simulink model "xpcFrameloop"  (Simulink 5.0)
settings: Solver=FixedStepDiscrete  StartTime=0.0  StopTime=10.0  RelTol=1e-3
libraries: dspsigattribs x2, xpclib x1, dspsrcs4 x1
settings Model: Creator=gweast  LastModifiedBy=gweast  ExtModeMexFile=ext_xpc  ExtModeArmWhenConnect=off  BooleanDataType=off  OptimizeBlockIOStorage=off  RTWSystemTargetFile=xpctarget.tlc  RTWTemplateMakefile=xpc_default_tmf  RTWOptions="-aEnforceIntegerDowncast=0 -aExtMode=1 -aFoldNonRolledExpr=0 -aForceParamTrailComments=0 -aGenerateComments=1 -aGenerateReport=0 -aIncDataTypeInIds=0 -aIncHierarchyInIds=0 -aInlineInvariantSignals=0 -aInlineParameters=0 -aInlinedPrmAccess=\"Literals\" -aLocalBlockOutputs=0 -aMaxRTWIdLen=31 -aPrefixModelToSubsysFcnNames=1 -aRL32IRQSourceModifier=\"Timer\" -aRL32LogBufSizeModifier=100000 -aRL32LogTETModifier=1 -aRL32ModeModifier=\"Real-Time\" -aRL32ObjectName=\"tg\" -aRTWVerbose=1 -aRollThreshold=5 -aShowEliminatedStatements=1 -axPCIOIRQSlot=-1 -axPCIRQSourceBoard=\"None/Other\" -axpcDblBuff=0 -axpcObjCom=0"

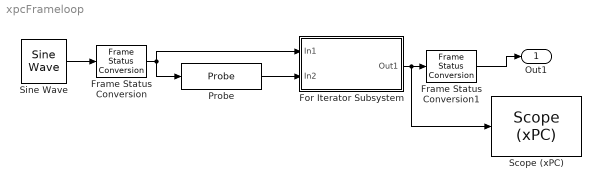
== system xpcFrameloop ==
  For Iterator Subsystem : Subsystem  TreatAsAtomicUnit=on
  Frame Status Conversion : dspsigattribs/Frame Status Conversion  growRefPort=off  outframe=Sample-based
  Frame Status Conversion1 : dspsigattribs/Frame Status Conversion  growRefPort=off  outframe=Frame-based
  Probe : Probe  ProbeSampleTime=off  ProbeComplexSignal=off
  "Scope (xPC) " : xpclib/Misc./Scope (xPC)   scopeno=1  scopetype=Target  viewmode=Graphical redraw  grid=on  ylimits=[0,0]  autostart=on  nosamples=100  noprepostsamples=0  interleave=1  triggermode=FreeRun  triggersignal=1  triggerlevel=0.0  triggerslope=either  triggerscope=1  triggersample=0
  Sine Wave : dspsrcs4/Sine Wave  Amplitude=1  Frequency=100  Phase=0  SampleMode=Discrete  OutComplex=Real  CompMethod=Trigonometric fcn  TableSize=Speed  SampleTime=1/1000  SamplesPerFrame=11  dataType=double  wordLen=16  udDataType=sfix(16)  fracBitsMode=Best precision  numFracBits=14  ResetState=Restart at time zero
  Out1 : Outport
  wires:
  Frame Status Conversion/1 -> For Iterator Subsystem/1(In1), Probe/1
  For Iterator Subsystem/1(Out1) -> Frame Status Conversion1/1, "Scope (xPC) "/1
  Frame Status Conversion1/1 -> Out1/1
  Probe/1 -> For Iterator Subsystem/2(In2)
  Sine Wave/1 -> Frame Status Conversion/1

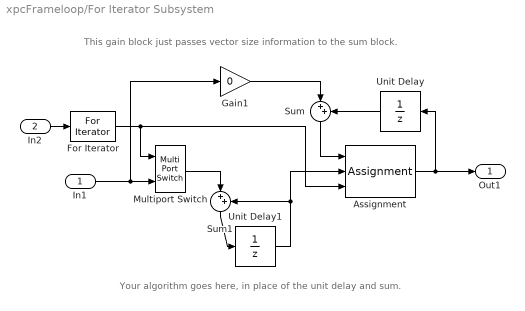
== system xpcFrameloop/For Iterator Subsystem ==
  note: Your algorithm goes here, in place of the
      | unit delay and sum.
  note: This gain block just passes vector
      | size information to the sum block.
  In1 : Inport
  In2 : Inport  Port=2
  Assignment : Assignment  ElementSrc=External
  For Iterator : ForIterator  IterationSource=external  NumIters=10
  Gain1 : Gain  Gain=0  SaturateOnIntegerOverflow=on
  Multiport Switch : MultiPortSwitch  Inputs=1  SaturateOnIntegerOverflow=on  InputSameDT=on
  Sum : Sum  Orientation=down  Inputs=|++  SaturateOnIntegerOverflow=on  InputSameDT=on
  Sum1 : Sum  Orientation=down  Inputs=|++  SaturateOnIntegerOverflow=on  InputSameDT=on
  Unit Delay : UnitDelay  Orientation=left  SampleTime=-1
  Unit Delay1 : UnitDelay  SampleTime=-1
  Out1 : Outport
  wires:
  For Iterator/1 -> Multiport Switch/1, Assignment/3
  In1/1 -> Multiport Switch/2, Gain1/1
  Assignment/1 -> Unit Delay/1, Out1/1
  Unit Delay1/1 -> Assignment/2, Sum1/2
  Unit Delay/1 -> Sum/2
  Sum/1 -> Assignment/1
  Gain1/1 -> Sum/1
  Multiport Switch/1 -> Sum1/1
  In2/1 -> For Iterator/1
  Sum1/1 -> Unit Delay1/1
